simulink model "third_RRR_robot_controller"  (R2018b)
settings: Solver=VariableStepAuto  StartTime=0.0  StopTime=10.0  RelTol=1e-3
libraries: roblocks x4
settings Model: Creator=aigerim.keutayeva  LastModifiedBy=aigerim.keutayeva

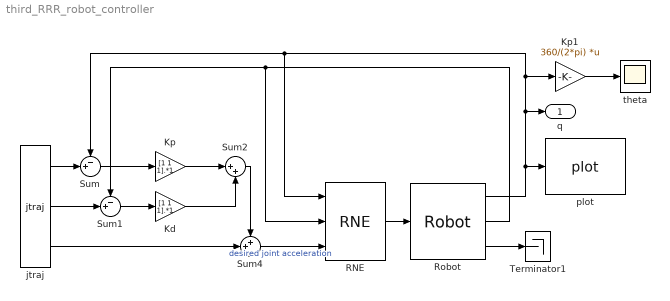
== system third_RRR_robot_controller ==
  Kd : Gain  Gain=[1 1 1].*1  SaturateOnIntegerOverflow=on  OutDataTypeStr=Inherit: Same as input  ParamDataTypeStr=Inherit: Same as input
  Kp : Gain  Gain=[1 1 1].*1  SaturateOnIntegerOverflow=on  OutDataTypeStr=Inherit: Same as input  ParamDataTypeStr=Inherit: Same as input
  Kp1 : Gain  Gain=360/(2*pi)  Multiplication=Matrix(K*u)  SaturateOnIntegerOverflow=on  OutDataTypeStr=Inherit: Same as input  ParamDataTypeStr=Inherit: Same as input
  RNE : roblocks/Arm/RNE  robot=RRR_robot  grav=[0 0 9.81]
  Robot : roblocks/Arm/Robot  robot=RRR_robot  q0=[0 0 0]
  Sum : Sum  Inputs=-+|  SaturateOnIntegerOverflow=on  InputSameDT=on  OutDataTypeStr=Inherit: Same as first input
  Sum1 : Sum  Inputs=-+|  SaturateOnIntegerOverflow=on  InputSameDT=on  OutDataTypeStr=Inherit: Same as first input
  Sum2 : Sum  Inputs=|++  SaturateOnIntegerOverflow=on  InputSameDT=on  OutDataTypeStr=Inherit: Same as first input
  Sum4 : Sum  Inputs=++|  SaturateOnIntegerOverflow=on  InputSameDT=on  OutDataTypeStr=Inherit: Same as first input
  Terminator1 : Terminator
  jtraj : roblocks/Toolbox/jtraj  q0=[0 0 0]  qf=[pi/2 -pi/4 -pi/4]  tmax=2  ts=0.02
  plot : roblocks/Arm/plot  robot=RRR_robot  fps=5  holdplot=on
  theta : Scope
  q : Outport
  wires:
  Robot/1 -> Kp1/1, Sum/1, RNE/1, q/1, plot/1
  jtraj/1 -> Sum/2
  jtraj/2 -> Sum1/2
  Robot/3 -> Terminator1/1
  Sum/1 -> Kp/1
  Sum1/1 -> Kd/1
  Kp/1 -> Sum2/1
  Kd/1 -> Sum2/2
  jtraj/3 -> Sum4/2
  Sum2/1 -> Sum4/1
  Sum4/1 -> RNE/3  "desired joint acceleration"
  Robot/2 -> RNE/2, Sum1/1
  RNE/1 -> Robot/1
  Kp1/1 -> theta/1
